simulink model "plant"  (R2024b)
settings: Solver=VariableStepAuto  StartTime=0.0  StopTime=20  RelTol=1e-3
undefined symbols (not defined in the file): Earth, init, Ts, Vehicle, WGS84
libraries: slpidlib x6, environmentLibrary x2, shared6dof x1, aerolibtransform2 x1
settings Model: Creator=Gabriel Fernandes  LastModifiedBy=Gabriel Fernandes

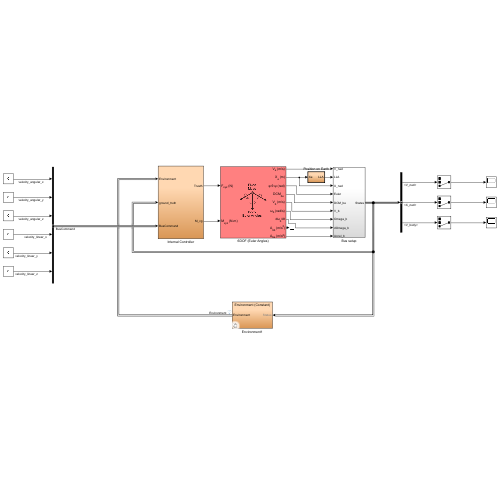
[thumbnail: Simulink's stored preview of the top-level diagram]
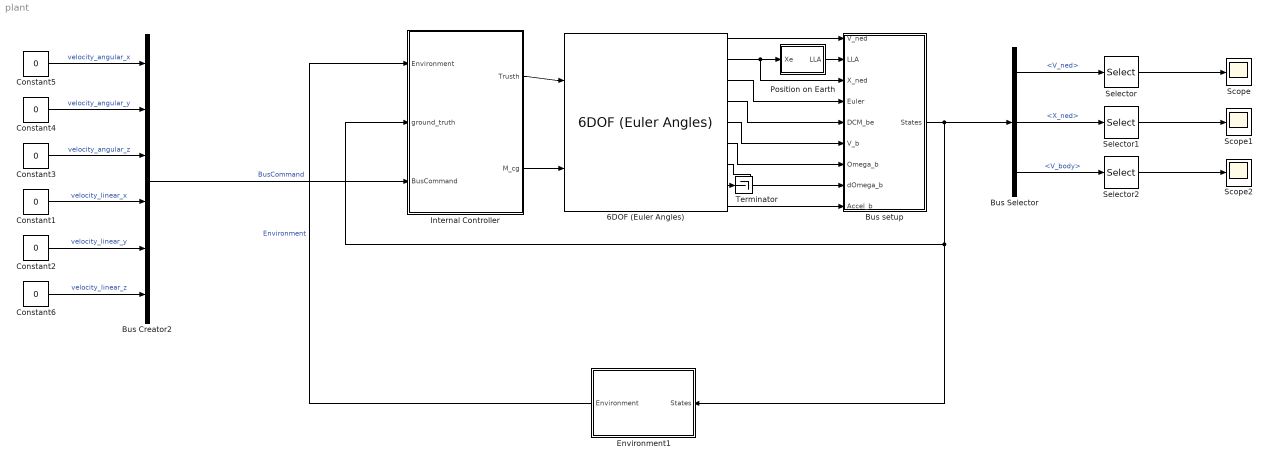
== system plant ==
  6DOF (Euler Angles) : shared6dof/6DOF (Euler Angles)  units=Metric (MKS)  mtype=Fixed  rep=Euler Angles  xme_0=init.posNED  Vm_0=init.vb  eul_0=init.euler  pm_0=init.angRates  mass_0=Vehicle.Airframe.mass  mass_e=0.5  mass_f=2.0  inertia=Vehicle.Airframe.inertia  inertia_e=eye(3)  inertia_f=2*eye(3)  k_quat=Vehicle.SixDOF.quatGain  vre_flag=on  abi_flag=on  aMode=aMode  xme_statename=''  Vm_statename=''  eul_statename=''  quat_statename=''  pm_statename=''  mass_statename=''
  Bus Creator2 : BusCreator  Inputs=6  OutDataTypeStr=Bus: BusCommand
  Bus Selector : BusSelector  OutputSignals=V_ned,X_ned,V_body
  Bus setup : Subsystem
  Constant{1..6} (6 alike) : Constant  Value=0
  Environment1 : Subsystem  Variant=on
  Internal Controller : Subsystem
  Position on Earth : Subsystem  Priority=1  TreatAsAtomicUnit=on
  Scope : Scope
  Scope1 : Scope
  Scope2 : Scope
  Selector : Selector  InputPortWidth=3  IndexOptions=Index vector (dialog)  Indices=3  OutputSizes=1
  Selector1 : Selector  InputPortWidth=3  IndexOptions=Index vector (dialog)  Indices=3  OutputSizes=1
  Selector2 : Selector  InputPortWidth=3  IndexOptions=Index vector (dialog)  Indices=3  OutputSizes=1
  Terminator : Terminator
  wires:
  6DOF (Euler Angles)/5 -> Bus setup/6(V_b)
  6DOF (Euler Angles)/2 -> Bus setup/3(X_ned), Position on Earth/1(Xe)
  6DOF (Euler Angles)/8 -> Terminator/1
  6DOF (Euler Angles)/6 -> Bus setup/7(Omega_b)
  6DOF (Euler Angles)/3 -> Bus setup/4(Euler)
  Position on Earth/1(LLA) -> Bus setup/2(LLA)
  6DOF (Euler Angles)/1 -> Bus setup/1(V_ned)
  6DOF (Euler Angles)/7 -> Bus setup/8(dOmega_b)
  6DOF (Euler Angles)/9 -> Bus setup/9(Accel_b)
  6DOF (Euler Angles)/4 -> Bus setup/5(DCM_be)
  Internal Controller/1(Trusth) -> 6DOF (Euler Angles)/1
  Internal Controller/2(M_cg) -> 6DOF (Euler Angles)/2
  Bus setup/1(States) -> Environment1/1(States), Internal Controller/2(ground_truth), Bus Selector/1
  Environment1/1(Environment) -> Internal Controller/1(Environment)  "Environment"
  Constant3/1 -> Bus Creator2/3  "velocity_angular_z"
  Constant5/1 -> Bus Creator2/1  "velocity_angular_x"
  Constant4/1 -> Bus Creator2/2  "velocity_angular_y"
  Constant1/1 -> Bus Creator2/4  "velocity_linear_x"
  Constant2/1 -> Bus Creator2/5  "velocity_linear_y"
  Constant6/1 -> Bus Creator2/6  "velocity_linear_z"
  Bus Creator2/1 -> Internal Controller/3(BusCommand)  "BusCommand"
  Bus Selector/1 -> Selector/1  "<V_ned>"
  Bus Selector/2 -> Selector1/1  "<X_ned>"
  Bus Selector/3 -> Selector2/1  "<V_body>"
  Selector/1 -> Scope/1
  Selector1/1 -> Scope1/1
  Selector2/1 -> Scope2/1

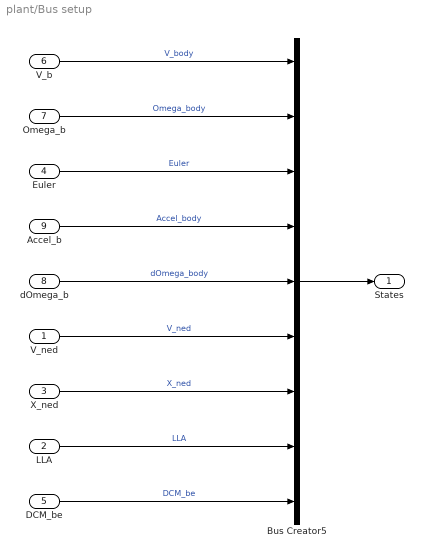
== system plant/Bus setup ==
  V_ned : Inport  Unit=m/second  PortDimensions=3
  LLA : Inport  Port=2  PortDimensions=3
  X_ned : Inport  Port=3  Unit=m  PortDimensions=3
  Euler : Inport  Port=4  Unit=rad  PortDimensions=3
  DCM_be : Inport  Port=5  PortDimensions=[3 3]
  V_b : Inport  Port=6  Unit=m/s  PortDimensions=3
  Omega_b : Inport  Port=7  Unit=rad/s  PortDimensions=3
  dOmega_b : Inport  Port=8  Unit=rad/s^2  PortDimensions=3
  Accel_b : Inport  Port=9  Unit=m/s^2  PortDimensions=3
  Bus Creator5 : BusCreator  Inputs=9  OutDataTypeStr=Bus: StatesBus  NonVirtualBus=on
  States : Outport  VectorParamsAs1DForOutWhenUnconnected=off
  wires:
  Bus Creator5/1 -> States/1
  V_b/1 -> Bus Creator5/1  "V_body"
  Omega_b/1 -> Bus Creator5/2  "Omega_body"
  Euler/1 -> Bus Creator5/3  "Euler"
  X_ned/1 -> Bus Creator5/7  "X_ned"
  Accel_b/1 -> Bus Creator5/4  "Accel_body"
  LLA/1 -> Bus Creator5/8  "LLA"
  dOmega_b/1 -> Bus Creator5/5  "dOmega_body"
  DCM_be/1 -> Bus Creator5/9  "DCM_be"
  V_ned/1 -> Bus Creator5/6  "V_ned"

== system plant/Environment1 ==
  note: VSS_ENVIRONMENT = 0 will select constant environment variables
      | VSS_ENVIRONMENT = 1 will select environment variables depending on position
  States : Inport  OutDataTypeStr=Bus: StatesBus
  Environment (Constant) : environmentLibrary/Environment (Constant)  SystemSampleTime=-1  VariantControl=VSS_ENVIRONMENT==EnvironmentMode.Constant  VariantActivationTime=update diagram  AllowFlexibleInterface=on  Latency=0  AutoFrameSizeCalculation=off
  Environment (Variable) : environmentLibrary/Environment (Variable)  SystemSampleTime=-1  VariantControl=VSS_ENVIRONMENT==EnvironmentMode.Variable  VariantActivationTime=update diagram  AllowFlexibleInterface=on  Latency=0  AutoFrameSizeCalculation=off
  Environment : Outport  OutDataTypeStr=Bus: EnvironmentBus  VectorParamsAs1DForOutWhenUnconnected=off

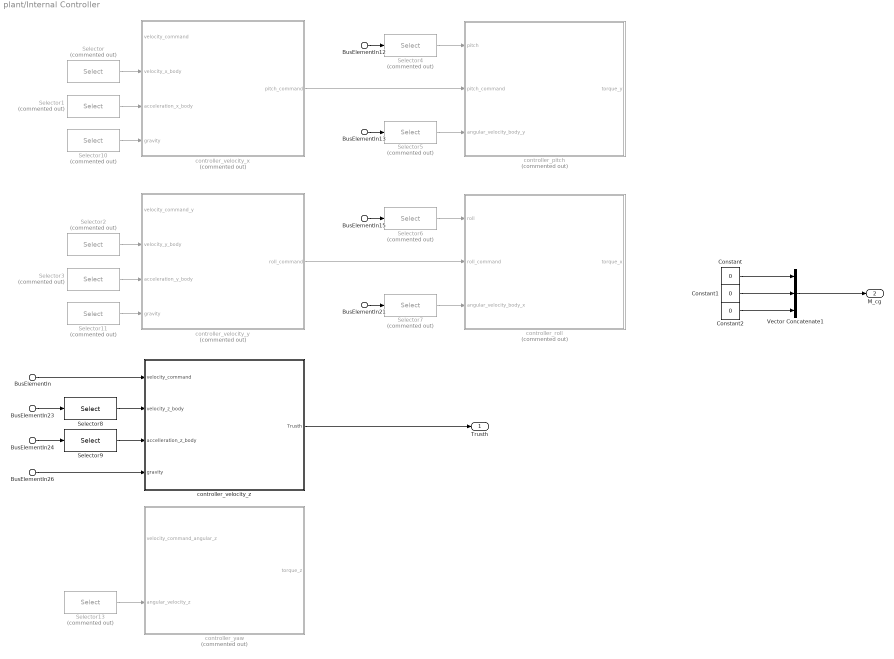
== system plant/Internal Controller ==
  BusElementIn26 : Inport  PortName=Environment  Element=Gravity_ned
  BusElementIn23 : Inport  Port=2  PortName=ground_truth  Element=V_body
  BusElementIn13 : Inport  Port=2  PortName=ground_truth  Element=Omega_body
  BusElementIn12 : Inport  Port=2  PortName=ground_truth  Element=Euler
  BusElementIn15 : Inport  Port=2  PortName=ground_truth  Element=Euler
  BusElementIn21 : Inport  Port=2  PortName=ground_truth  Element=Accel_body
  BusElementIn24 : Inport  Port=2  PortName=ground_truth  Element=Accel_body
  BusElementIn : Inport  Port=3  PortName=BusCommand  Element=velocity_linear_z
  Constant : Constant  Value=0
  Constant1 : Constant  Value=0
  Constant2 : Constant  Value=0
  Selector{,1,6..7} (4 alike) : Selector  Commented=on  InputPortWidth=3  IndexOptions=Index vector (dialog)  Indices=1  OutputSizes=1
  Selector10 : Selector  Commented=on  InputPortWidth=3  IndexOptions=Index vector (dialog)  Indices=3  OutputSizes=1
  Selector11 : Selector  Commented=on  InputPortWidth=3  IndexOptions=Index vector (dialog)  Indices=3  OutputSizes=1
  Selector13 : Selector  Commented=on  InputPortWidth=3  IndexOptions=Index vector (dialog)  Indices=3  OutputSizes=1
  Selector{2..5} (4 alike) : Selector  Commented=on  InputPortWidth=3  IndexOptions=Index vector (dialog)  Indices=2  OutputSizes=1
  Selector8 : Selector  InputPortWidth=3  IndexOptions=Index vector (dialog)  Indices=3  OutputSizes=1
  Selector9 : Selector  InputPortWidth=3  IndexOptions=Index vector (dialog)  Indices=3  OutputSizes=1
  Vector Concatenate1 : Concatenate  NumInputs=3
  controller_pitch : Subsystem  Commented=on
  controller_roll : Subsystem  Commented=on
  controller_velocity_x : Subsystem  Commented=on
  controller_velocity_y : Subsystem  Commented=on
  controller_velocity_z : Subsystem
  controller_yaw : Subsystem  Commented=on
  Trusth : Outport  Unit=N  VectorParamsAs1DForOutWhenUnconnected=off
  M_cg : Outport  Port=2  Unit=N*m  VectorParamsAs1DForOutWhenUnconnected=off
  wires:
  Vector Concatenate1/1 -> M_cg/1
  ? -> Selector/1
  Selector/1 -> controller_velocity_x/2(velocity_x_body)
  ? -> Selector1/1
  Selector1/1 -> controller_velocity_x/3(acceleration_x_body)
  ? -> Selector10/1
  ? -> Selector3/1
  ? -> Selector2/1
  Selector2/1 -> controller_velocity_y/2(velocity_y_body)
  Selector3/1 -> controller_velocity_y/3(acceleration_y_body)
  ? -> Selector11/1
  controller_velocity_x/1(pitch_command) -> controller_pitch/2(pitch_command)
  BusElementIn12/1 -> Selector4/1
  Selector4/1 -> controller_pitch/1(pitch)
  BusElementIn13/1 -> Selector5/1
  Selector5/1 -> controller_pitch/3(angular_velocity_body_y)
  Selector7/1 -> controller_roll/3(angular_velocity_body_x)
  Selector6/1 -> controller_roll/1(roll)
  controller_velocity_y/1(roll_command) -> controller_roll/2(roll_command)
  BusElementIn15/1 -> Selector6/1
  BusElementIn21/1 -> Selector7/1
  BusElementIn23/1 -> Selector8/1
  Selector8/1 -> controller_velocity_z/2(velocity_z_body)
  BusElementIn24/1 -> Selector9/1
  Selector9/1 -> controller_velocity_z/3(accelleration_z_body)
  Selector10/1 -> controller_velocity_x/4(gravity)
  Selector11/1 -> controller_velocity_y/4(gravity)
  BusElementIn26/1 -> controller_velocity_z/4(gravity)
  Selector13/1 -> controller_yaw/2(angular_velocity_z)
  controller_velocity_z/1(Trusth) -> Trusth/1
  BusElementIn/1 -> controller_velocity_z/1(velocity_command)
  Constant/1 -> Vector Concatenate1/1
  Constant1/1 -> Vector Concatenate1/2
  Constant2/1 -> Vector Concatenate1/3

== system plant/Position on Earth ==
  Xe : Inport  Unit=m
  Flat Earth to LLA : aerolibtransform2/Flat Earth to LLA  units=Metric (MKS)  ptype=Earth (WGS84)  F=1/298.257223563  R=6378137  refPosPort=off  LL0=init.posLLA(1:2)  psi=Vehicle.PositionOnEarth.FlatEarthToLLA.xAxis
  Mux : Mux  Inputs=2
  href : Constant  Value=Vehicle.PositionOnEarth.href
  LLA : Outport  VectorParamsAs1DForOutWhenUnconnected=off
  wires:
  Mux/1 -> LLA/1
  Xe/1 -> Flat Earth to LLA/1
  Flat Earth to LLA/1 -> Mux/1
  Flat Earth to LLA/2 -> Mux/2
  href/1 -> Flat Earth to LLA/2

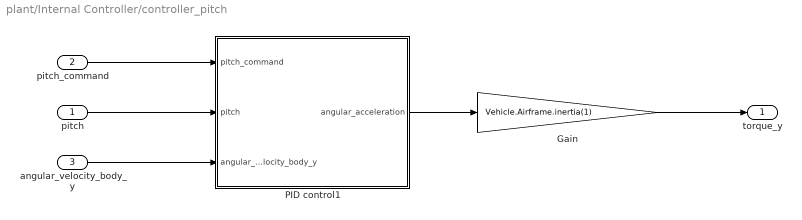
== system plant/Internal Controller/controller_pitch ==
  pitch : Inport
  pitch_command : Inport  Port=2
  angular_velocity_body_y : Inport  Port=3
  Gain : Gain  Gain=Vehicle.Airframe.inertia(1)
  PID control1 : Subsystem
  torque_y : Outport
  wires:
  pitch_command/1 -> PID control1/1(pitch_command)
  pitch/1 -> PID control1/2(pitch)
  angular_velocity_body_y/1 -> PID control1/3(angular_velocity_body_y)
  PID control1/1(angular_acceleration) -> Gain/1
  Gain/1 -> torque_y/1

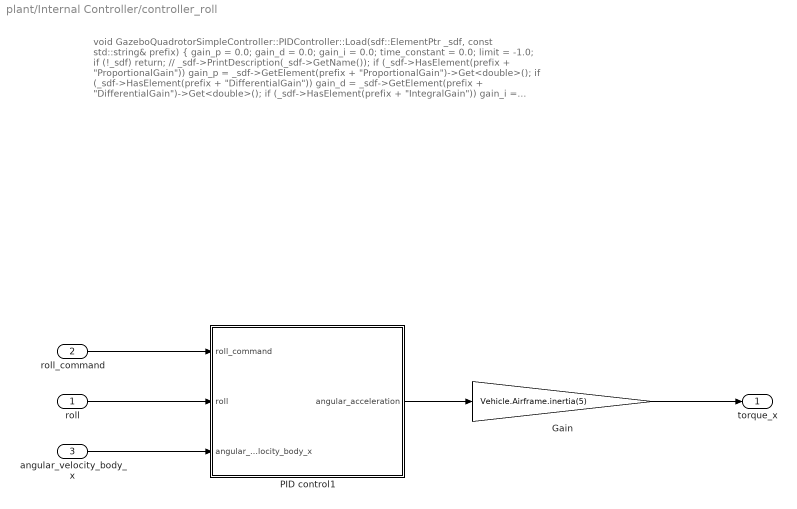
== system plant/Internal Controller/controller_roll ==
  note: void GazeboQuadrotorSimpleController::PIDController::Load(sdf::ElementPtr _sdf, const std::string& prefix)
      | {
      |   gain_p = 0.0;
      |   gain_d = 0.0;
      |   gain_i = 0.0;
      |   time_constant = 0.0;
      |   limit = -1.0;
      |
      |   if (!_sdf) return;
      |   // _sdf->PrintDescription(_sdf->GetName());
      |   if (_sdf->HasElement(prefix + "ProportionalGain")) gain_p = _sdf->GetElement(prefix + "ProportionalGain")->Get<double>();
      |   if (_sdf->HasElement(prefix + "DifferentialGain")) gain_d = _sdf->GetElement(prefix + "DifferentialGain")->Get<double>();
      |   if (_sdf->HasElement(prefix + "IntegralGain"))     gain_i = _sdf->GetElement(prefix + "IntegralGain")->Get<double>();
      |   if (_sdf->HasElement(prefix + "TimeConstant"))     time_constant = _sdf->GetElement(prefix + "TimeConstant")->Get<double>();
      |   if (_sdf->HasElement(prefix + "Limit"))            limit = _sdf->GetElement(prefix + "Limit")->Get<double>();
      | }
  roll : Inport
  roll_command : Inport  Port=2
  angular_velocity_body_x : Inport  Port=3
  Gain : Gain  Gain=Vehicle.Airframe.inertia(5)
  PID control1 : Subsystem
  torque_x : Outport
  wires:
  roll_command/1 -> PID control1/1(roll_command)
  roll/1 -> PID control1/2(roll)
  angular_velocity_body_x/1 -> PID control1/3(angular_velocity_body_x)
  PID control1/1(angular_acceleration) -> Gain/1
  Gain/1 -> torque_x/1

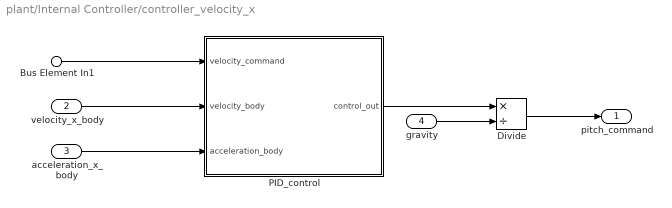
== system plant/Internal Controller/controller_velocity_x ==
  Bus Element In1 : Inport  PortName=velocity_command
  velocity_x_body : Inport  Port=2
  acceleration_x_body : Inport  Port=3
  gravity : Inport  Port=4
  Divide : Product  Inputs=*/
  PID_control : Subsystem
  pitch_command : Outport
  wires:
  velocity_x_body/1 -> PID_control/2(velocity_body)
  acceleration_x_body/1 -> PID_control/3(acceleration_body)
  PID_control/1(control_out) -> Divide/1
  Divide/1 -> pitch_command/1
  gravity/1 -> Divide/2
  Bus Element In1/1 -> PID_control/1(velocity_command)

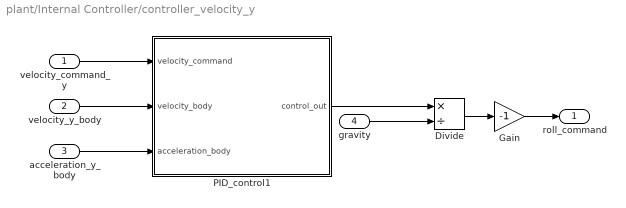
== system plant/Internal Controller/controller_velocity_y ==
  velocity_command_y : Inport
  velocity_y_body : Inport  Port=2
  acceleration_y_body : Inport  Port=3
  gravity : Inport  Port=4
  Divide : Product  Inputs=*/
  Gain : Gain  Gain=-1
  PID_control1 : Subsystem
  roll_command : Outport
  wires:
  PID_control1/1(control_out) -> Divide/1
  gravity/1 -> Divide/2
  velocity_command_y/1 -> PID_control1/1(velocity_command)
  velocity_y_body/1 -> PID_control1/2(velocity_body)
  acceleration_y_body/1 -> PID_control1/3(acceleration_body)
  Divide/1 -> Gain/1
  Gain/1 -> roll_command/1

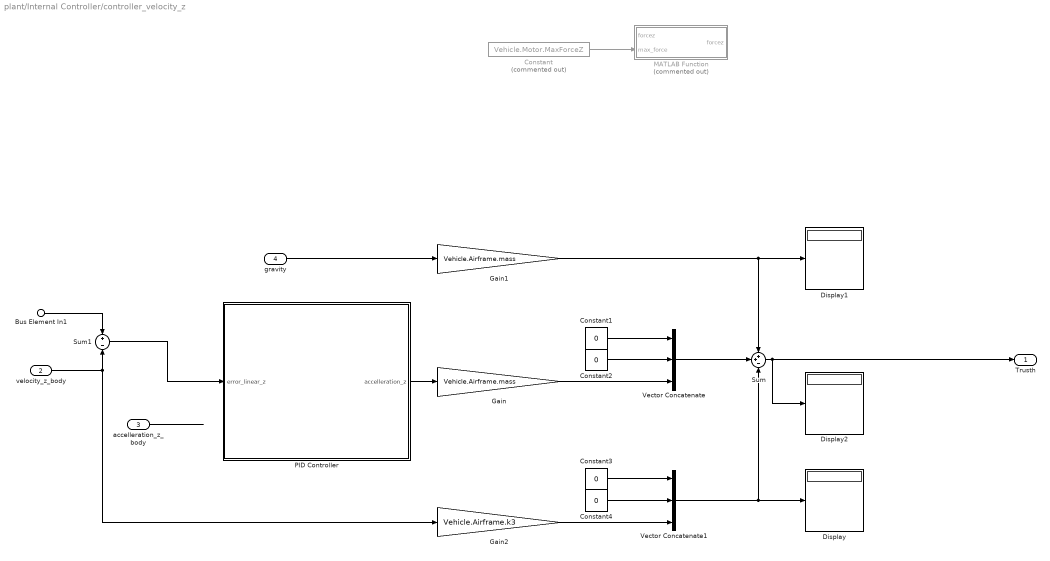
== system plant/Internal Controller/controller_velocity_z ==
  Bus Element In1 : Inport  PortName=velocity_command
  velocity_z_body : Inport  Port=2
  accelleration_z_body : Inport  Port=3
  gravity : Inport  Port=4
  Constant : Constant  Commented=on  Value=Vehicle.Motor.MaxForceZ
  Constant{1..4} (4 alike) : Constant  Value=0
  Display : Display
  Display1 : Display
  Display2 : Display
  Gain : Gain  Gain=Vehicle.Airframe.mass
  Gain1 : Gain  Gain=Vehicle.Airframe.mass
  Gain2 : Gain  Gain=Vehicle.Airframe.k3
  MATLAB Function : MATLAB Function  Commented=on  TreatAsAtomicUnit=on
  PID Controller : Subsystem
  Sum : Sum  Inputs=++-
  Sum1 : Sum  Inputs=+-
  Vector Concatenate : Concatenate  NumInputs=3
  Vector Concatenate1 : Concatenate  NumInputs=3
  Trusth : Outport
  wires:
  Sum/1 -> Display2/1, Trusth/1
  gravity/1 -> Gain1/1
  Bus Element In1/1 -> Sum1/1
  velocity_z_body/1 -> Gain2/1, Sum1/2
  accelleration_z_body/1 -> ?
  PID Controller/1(accelleration_z) -> Gain/1
  Gain1/1 -> Sum/1, Display1/1
  Gain/1 -> Vector Concatenate/3
  Vector Concatenate/1 -> Sum/2
  Constant1/1 -> Vector Concatenate/1
  Constant2/1 -> Vector Concatenate/2
  ? -> MATLAB Function/1("forcez ")
  Constant/1 -> MATLAB Function/2(max_force)
  Gain2/1 -> Vector Concatenate1/3
  Sum1/1 -> PID Controller/1(error_linear_z)
  Constant3/1 -> Vector Concatenate1/1
  Constant4/1 -> Vector Concatenate1/2
  Vector Concatenate1/1 -> Display/1, Sum/3

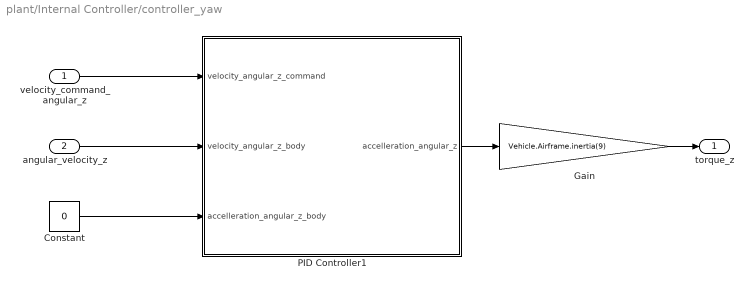
== system plant/Internal Controller/controller_yaw ==
  velocity_command_angular_z : Inport
  angular_velocity_z : Inport  Port=2
  Constant : Constant  Value=0
  Gain : Gain  Gain=Vehicle.Airframe.inertia(9)
  PID Controller1 : Subsystem
  torque_z : Outport
  wires:
  velocity_command_angular_z/1 -> PID Controller1/1(velocity_angular_z_command)
  angular_velocity_z/1 -> PID Controller1/2(velocity_angular_z_body)
  Constant/1 -> PID Controller1/3(accelleration_angular_z_body)
  PID Controller1/1(accelleration_angular_z) -> Gain/1
  Gain/1 -> torque_z/1

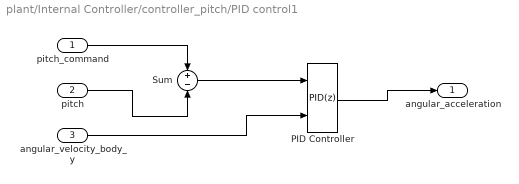
== system plant/Internal Controller/controller_pitch/PID control1 ==
  pitch_command : Inport
  pitch : Inport  Port=2
  angular_velocity_body_y : Inport  Port=3
  PID Controller : slpidlib/PID Controller  Controller=PID  Form=Parallel  TimeDomain=Discrete-time  UseExternalTs=off  SampleTime=Ts  IntegratorMethod=Forward Euler  FilterMethod=Forward Euler  ControllerParametersSource=internal  P=1  I=1  UseKiTs=off  D=0  UseExternalDerivativeSource=on  N=100  UseFilter=on  TunerSelectOption=Transfer Function Based (PID Tuner App)  InitialConditionSource=internal  InitialConditionForIntegrator=0  InitialConditionForFilter=0  DifferentiatorICPrevScaledInput=0  ExternalReset=none  TrackingMode=off  Kt=1  LimitOutput=off  SatLimitsSource=internal  UpperSaturationLimit=inf  LowerSaturationLimit=-inf  LinearizeAsGain=on  AntiWindupMode=none  Kb=1  LimitIntegrator=off  UpperIntegratorSaturationLimit=inf  LowerIntegratorSaturationLimit=-inf  POutMin=[]  POutMax=[]  IOutMin=[]  IOutMax=[]  DOutMin=[]  DOutMax=[]  NOutMin=[]  NOutMax=[]  SumOutMin=[]  SumOutMax=[]  SaturationOutMin=[]  SaturationOutMax=[]  PParamMin=[]  PParamMax=[]  IParamMin=[]  IParamMax=[]  DParamMin=[]  DParamMax=[]  NParamMin=[]  NParamMax=[]  KbParamMin=[]  KbParamMax=[]  KtParamMin=[]  KtParamMax=[]  KbOutMin=[]  KbOutMax=[]  KtOutMin=[]  KtOutMax=[]  IntegratorOutMin=[]  IntegratorOutMax=[]  FilterOutMin=[]  FilterOutMax=[]  SumI1OutMin=[]  SumI1OutMax=[]  SumI2OutMin=[]  SumI2OutMax=[]  SumI3OutMin=[]  SumI3OutMax=[]  SumI4OutMin=[]  SumI4OutMax=[]  SumDOutMin=[]  SumDOutMax=[]  DifferentiatorOutMin=[]  DifferentiatorOutMax=[]  FilterDiffOutCoefMin=[]  FilterDiffOutCoefMax=[]  ReciprocalOutMin=[]  ReciprocalOutMax=[]  SumDenOutMin=[]  SumDenOutMax=[]  SumNumOutMin=[]  SumNumOutMax=[]  DivideOutMin=[]  DivideOutMax=[]  UdiffTsProdOutMin=[]  UdiffTsProdOutMax=[]  NTsProdOutMin=[]  NTsProdOutMax=[]  UintegralTsProdOutMin=[]  UintegralTsProdOutMax=[]  UngainTsProdOutMin=[]  UngainTsProdOutMax=[]  ClampingZeroOutDataTypeStr=Inherit: Inherit via back propagation  ClampingZeroOutMin=[]  ClampingZeroOutMax=[]  FilterDenConstantOutDataTypeStr=Inherit: Inherit via back propagation  FilterDenConstantOutMin=[]  FilterDenConstantOutMax=[]  PCopyOutDataTypeStr=Inherit: Inherit via back propagation  PCopyOutMin=[]  PCopyOutMax=[]  NCopyOutDataTypeStr=Inherit: Inherit via back propagation  NCopyOutMin=[]  NCopyOutMax=[]  IntegratorContinuousStateAttributes=''  IntegratorStateMustResolveToSignalObject=off  IntegratorRTWStateStorageClass=Auto  FilterContinuousStateAttributes=''  FilterStateMustResolveToSignalObject=off  FilterRTWStateStorageClass=Auto  ParallelPVariant=InternalParameters  IdealPVariant=Disabled  IVariant=InternalParameters  DVariant=InternalParameters  IntegratorVariant=Discrete  SatVariant=Disabled  AWVariant=Passthrough  PCopyVariant=Disabled  TRVariant=Disabled  FdbkBlocksVariant=Forward  IdealPFdbkVariant=Disabled  SatFdbkVariant=Disabled  DerivativeFilterVariant=ForwardEulerFilterOnly  NVariant=InternalParameters  NCopyVariant=Disabled  FilterICVariant=InternalICsFilter  IntegratorICVariant=InternalICs  ExternalResetVariant=Disabled  TRSumVariant=Passthrough  SumFdbkVariant=Disabled  SumVariant=Sum_PID  TsampFilterVariant=InternalTs  TsampNgainVariant=Passthrough  TsampIntegralVariant=Disabled_SignalSpec  ExternalSaturationOutDataTypeStr=Inherit: Same as second input  DerivativeSourceVariant=ExternalYdot  PreIntVariant=InternalPreInt
  Sum : Sum  Inputs=+-
  angular_acceleration : Outport
  wires:
  pitch/1 -> Sum/2
  pitch_command/1 -> Sum/1
  PID Controller/1 -> angular_acceleration/1
  Sum/1 -> PID Controller/1
  angular_velocity_body_y/1 -> PID Controller/2

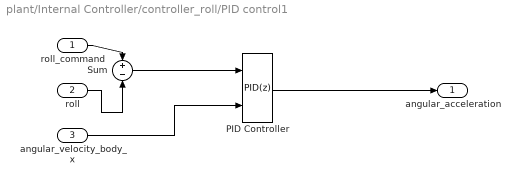
== system plant/Internal Controller/controller_roll/PID control1 ==
  roll_command : Inport
  roll : Inport  Port=2
  angular_velocity_body_x : Inport  Port=3
  PID Controller : slpidlib/PID Controller  Controller=PID  Form=Parallel  TimeDomain=Discrete-time  UseExternalTs=off  SampleTime=Ts  IntegratorMethod=Forward Euler  FilterMethod=Forward Euler  ControllerParametersSource=internal  P=1  I=1  UseKiTs=off  D=0  UseExternalDerivativeSource=on  N=100  UseFilter=on  TunerSelectOption=Transfer Function Based (PID Tuner App)  InitialConditionSource=internal  InitialConditionForIntegrator=0  InitialConditionForFilter=0  DifferentiatorICPrevScaledInput=0  ExternalReset=none  TrackingMode=off  Kt=1  LimitOutput=off  SatLimitsSource=internal  UpperSaturationLimit=inf  LowerSaturationLimit=-inf  LinearizeAsGain=on  AntiWindupMode=none  Kb=1  LimitIntegrator=off  UpperIntegratorSaturationLimit=inf  LowerIntegratorSaturationLimit=-inf  POutMin=[]  POutMax=[]  IOutMin=[]  IOutMax=[]  DOutMin=[]  DOutMax=[]  NOutMin=[]  NOutMax=[]  SumOutMin=[]  SumOutMax=[]  SaturationOutMin=[]  SaturationOutMax=[]  PParamMin=[]  PParamMax=[]  IParamMin=[]  IParamMax=[]  DParamMin=[]  DParamMax=[]  NParamMin=[]  NParamMax=[]  KbParamMin=[]  KbParamMax=[]  KtParamMin=[]  KtParamMax=[]  KbOutMin=[]  KbOutMax=[]  KtOutMin=[]  KtOutMax=[]  IntegratorOutMin=[]  IntegratorOutMax=[]  FilterOutMin=[]  FilterOutMax=[]  SumI1OutMin=[]  SumI1OutMax=[]  SumI2OutMin=[]  SumI2OutMax=[]  SumI3OutMin=[]  SumI3OutMax=[]  SumI4OutMin=[]  SumI4OutMax=[]  SumDOutMin=[]  SumDOutMax=[]  DifferentiatorOutMin=[]  DifferentiatorOutMax=[]  FilterDiffOutCoefMin=[]  FilterDiffOutCoefMax=[]  ReciprocalOutMin=[]  ReciprocalOutMax=[]  SumDenOutMin=[]  SumDenOutMax=[]  SumNumOutMin=[]  SumNumOutMax=[]  DivideOutMin=[]  DivideOutMax=[]  UdiffTsProdOutMin=[]  UdiffTsProdOutMax=[]  NTsProdOutMin=[]  NTsProdOutMax=[]  UintegralTsProdOutMin=[]  UintegralTsProdOutMax=[]  UngainTsProdOutMin=[]  UngainTsProdOutMax=[]  ClampingZeroOutDataTypeStr=Inherit: Inherit via back propagation  ClampingZeroOutMin=[]  ClampingZeroOutMax=[]  FilterDenConstantOutDataTypeStr=Inherit: Inherit via back propagation  FilterDenConstantOutMin=[]  FilterDenConstantOutMax=[]  PCopyOutDataTypeStr=Inherit: Inherit via back propagation  PCopyOutMin=[]  PCopyOutMax=[]  NCopyOutDataTypeStr=Inherit: Inherit via back propagation  NCopyOutMin=[]  NCopyOutMax=[]  IntegratorContinuousStateAttributes=''  IntegratorStateMustResolveToSignalObject=off  IntegratorRTWStateStorageClass=Auto  FilterContinuousStateAttributes=''  FilterStateMustResolveToSignalObject=off  FilterRTWStateStorageClass=Auto  ParallelPVariant=InternalParameters  IdealPVariant=Disabled  IVariant=InternalParameters  DVariant=InternalParameters  IntegratorVariant=Discrete  SatVariant=Disabled  AWVariant=Passthrough  PCopyVariant=Disabled  TRVariant=Disabled  FdbkBlocksVariant=Forward  IdealPFdbkVariant=Disabled  SatFdbkVariant=Disabled  DerivativeFilterVariant=ForwardEulerFilterOnly  NVariant=InternalParameters  NCopyVariant=Disabled  FilterICVariant=InternalICsFilter  IntegratorICVariant=InternalICs  ExternalResetVariant=Disabled  TRSumVariant=Passthrough  SumFdbkVariant=Disabled  SumVariant=Sum_PID  TsampFilterVariant=InternalTs  TsampNgainVariant=Passthrough  TsampIntegralVariant=Disabled_SignalSpec  ExternalSaturationOutDataTypeStr=Inherit: Same as second input  DerivativeSourceVariant=ExternalYdot  PreIntVariant=InternalPreInt
  Sum : Sum  Inputs=+-
  angular_acceleration : Outport
  wires:
  roll/1 -> Sum/2
  roll_command/1 -> Sum/1
  PID Controller/1 -> angular_acceleration/1
  Sum/1 -> PID Controller/1
  angular_velocity_body_x/1 -> PID Controller/2

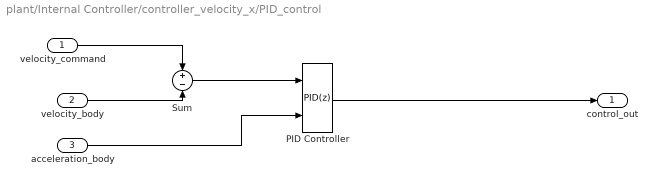
== system plant/Internal Controller/controller_velocity_x/PID_control ==
  velocity_command : Inport
  velocity_body : Inport  Port=2
  acceleration_body : Inport  Port=3
  PID Controller : slpidlib/PID Controller  Controller=PID  Form=Parallel  TimeDomain=Discrete-time  UseExternalTs=off  SampleTime=Ts  IntegratorMethod=Forward Euler  FilterMethod=Forward Euler  ControllerParametersSource=internal  P=1  I=1  UseKiTs=off  D=0  UseExternalDerivativeSource=on  N=100  UseFilter=on  TunerSelectOption=Transfer Function Based (PID Tuner App)  InitialConditionSource=internal  InitialConditionForIntegrator=0  InitialConditionForFilter=0  DifferentiatorICPrevScaledInput=0  ExternalReset=none  TrackingMode=off  Kt=1  LimitOutput=off  SatLimitsSource=internal  UpperSaturationLimit=inf  LowerSaturationLimit=-inf  LinearizeAsGain=on  AntiWindupMode=none  Kb=1  LimitIntegrator=off  UpperIntegratorSaturationLimit=inf  LowerIntegratorSaturationLimit=-inf  POutMin=[]  POutMax=[]  IOutMin=[]  IOutMax=[]  DOutMin=[]  DOutMax=[]  NOutMin=[]  NOutMax=[]  SumOutMin=[]  SumOutMax=[]  SaturationOutMin=[]  SaturationOutMax=[]  PParamMin=[]  PParamMax=[]  IParamMin=[]  IParamMax=[]  DParamMin=[]  DParamMax=[]  NParamMin=[]  NParamMax=[]  KbParamMin=[]  KbParamMax=[]  KtParamMin=[]  KtParamMax=[]  KbOutMin=[]  KbOutMax=[]  KtOutMin=[]  KtOutMax=[]  IntegratorOutMin=[]  IntegratorOutMax=[]  FilterOutMin=[]  FilterOutMax=[]  SumI1OutMin=[]  SumI1OutMax=[]  SumI2OutMin=[]  SumI2OutMax=[]  SumI3OutMin=[]  SumI3OutMax=[]  SumI4OutMin=[]  SumI4OutMax=[]  SumDOutMin=[]  SumDOutMax=[]  DifferentiatorOutMin=[]  DifferentiatorOutMax=[]  FilterDiffOutCoefMin=[]  FilterDiffOutCoefMax=[]  ReciprocalOutMin=[]  ReciprocalOutMax=[]  SumDenOutMin=[]  SumDenOutMax=[]  SumNumOutMin=[]  SumNumOutMax=[]  DivideOutMin=[]  DivideOutMax=[]  UdiffTsProdOutMin=[]  UdiffTsProdOutMax=[]  NTsProdOutMin=[]  NTsProdOutMax=[]  UintegralTsProdOutMin=[]  UintegralTsProdOutMax=[]  UngainTsProdOutMin=[]  UngainTsProdOutMax=[]  ClampingZeroOutDataTypeStr=Inherit: Inherit via back propagation  ClampingZeroOutMin=[]  ClampingZeroOutMax=[]  FilterDenConstantOutDataTypeStr=Inherit: Inherit via back propagation  FilterDenConstantOutMin=[]  FilterDenConstantOutMax=[]  PCopyOutDataTypeStr=Inherit: Inherit via back propagation  PCopyOutMin=[]  PCopyOutMax=[]  NCopyOutDataTypeStr=Inherit: Inherit via back propagation  NCopyOutMin=[]  NCopyOutMax=[]  IntegratorContinuousStateAttributes=''  IntegratorStateMustResolveToSignalObject=off  IntegratorRTWStateStorageClass=Auto  FilterContinuousStateAttributes=''  FilterStateMustResolveToSignalObject=off  FilterRTWStateStorageClass=Auto  ParallelPVariant=InternalParameters  IdealPVariant=Disabled  IVariant=InternalParameters  DVariant=InternalParameters  IntegratorVariant=Discrete  SatVariant=Disabled  AWVariant=Passthrough  PCopyVariant=Disabled  TRVariant=Disabled  FdbkBlocksVariant=Forward  IdealPFdbkVariant=Disabled  SatFdbkVariant=Disabled  DerivativeFilterVariant=ForwardEulerFilterOnly  NVariant=InternalParameters  NCopyVariant=Disabled  FilterICVariant=InternalICsFilter  IntegratorICVariant=InternalICs  ExternalResetVariant=Disabled  TRSumVariant=Passthrough  SumFdbkVariant=Disabled  SumVariant=Sum_PID  TsampFilterVariant=InternalTs  TsampNgainVariant=Passthrough  TsampIntegralVariant=Disabled_SignalSpec  ExternalSaturationOutDataTypeStr=Inherit: Same as second input  DerivativeSourceVariant=ExternalYdot  PreIntVariant=InternalPreInt
  Sum : Sum  Inputs=+-
  control_out : Outport
  wires:
  velocity_body/1 -> Sum/2
  velocity_command/1 -> Sum/1
  PID Controller/1 -> control_out/1
  Sum/1 -> PID Controller/1
  acceleration_body/1 -> PID Controller/2

== system plant/Internal Controller/controller_velocity_y/PID_control1 ==
  velocity_command : Inport
  velocity_body : Inport  Port=2
  acceleration_body : Inport  Port=3
  PID Controller : slpidlib/PID Controller  Controller=PID  Form=Parallel  TimeDomain=Discrete-time  UseExternalTs=off  SampleTime=Ts  IntegratorMethod=Forward Euler  FilterMethod=Forward Euler  ControllerParametersSource=internal  P=1  I=1  UseKiTs=off  D=0  UseExternalDerivativeSource=on  N=100  UseFilter=on  TunerSelectOption=Transfer Function Based (PID Tuner App)  InitialConditionSource=internal  InitialConditionForIntegrator=0  InitialConditionForFilter=0  DifferentiatorICPrevScaledInput=0  ExternalReset=none  TrackingMode=off  Kt=1  LimitOutput=off  SatLimitsSource=internal  UpperSaturationLimit=inf  LowerSaturationLimit=-inf  LinearizeAsGain=on  AntiWindupMode=none  Kb=1  LimitIntegrator=off  UpperIntegratorSaturationLimit=inf  LowerIntegratorSaturationLimit=-inf  POutMin=[]  POutMax=[]  IOutMin=[]  IOutMax=[]  DOutMin=[]  DOutMax=[]  NOutMin=[]  NOutMax=[]  SumOutMin=[]  SumOutMax=[]  SaturationOutMin=[]  SaturationOutMax=[]  PParamMin=[]  PParamMax=[]  IParamMin=[]  IParamMax=[]  DParamMin=[]  DParamMax=[]  NParamMin=[]  NParamMax=[]  KbParamMin=[]  KbParamMax=[]  KtParamMin=[]  KtParamMax=[]  KbOutMin=[]  KbOutMax=[]  KtOutMin=[]  KtOutMax=[]  IntegratorOutMin=[]  IntegratorOutMax=[]  FilterOutMin=[]  FilterOutMax=[]  SumI1OutMin=[]  SumI1OutMax=[]  SumI2OutMin=[]  SumI2OutMax=[]  SumI3OutMin=[]  SumI3OutMax=[]  SumI4OutMin=[]  SumI4OutMax=[]  SumDOutMin=[]  SumDOutMax=[]  DifferentiatorOutMin=[]  DifferentiatorOutMax=[]  FilterDiffOutCoefMin=[]  FilterDiffOutCoefMax=[]  ReciprocalOutMin=[]  ReciprocalOutMax=[]  SumDenOutMin=[]  SumDenOutMax=[]  SumNumOutMin=[]  SumNumOutMax=[]  DivideOutMin=[]  DivideOutMax=[]  UdiffTsProdOutMin=[]  UdiffTsProdOutMax=[]  NTsProdOutMin=[]  NTsProdOutMax=[]  UintegralTsProdOutMin=[]  UintegralTsProdOutMax=[]  UngainTsProdOutMin=[]  UngainTsProdOutMax=[]  ClampingZeroOutDataTypeStr=Inherit: Inherit via back propagation  ClampingZeroOutMin=[]  ClampingZeroOutMax=[]  FilterDenConstantOutDataTypeStr=Inherit: Inherit via back propagation  FilterDenConstantOutMin=[]  FilterDenConstantOutMax=[]  PCopyOutDataTypeStr=Inherit: Inherit via back propagation  PCopyOutMin=[]  PCopyOutMax=[]  NCopyOutDataTypeStr=Inherit: Inherit via back propagation  NCopyOutMin=[]  NCopyOutMax=[]  IntegratorContinuousStateAttributes=''  IntegratorStateMustResolveToSignalObject=off  IntegratorRTWStateStorageClass=Auto  FilterContinuousStateAttributes=''  FilterStateMustResolveToSignalObject=off  FilterRTWStateStorageClass=Auto  ParallelPVariant=InternalParameters  IdealPVariant=Disabled  IVariant=InternalParameters  DVariant=InternalParameters  IntegratorVariant=Discrete  SatVariant=Disabled  AWVariant=Passthrough  PCopyVariant=Disabled  TRVariant=Disabled  FdbkBlocksVariant=Forward  IdealPFdbkVariant=Disabled  SatFdbkVariant=Disabled  DerivativeFilterVariant=ForwardEulerFilterOnly  NVariant=InternalParameters  NCopyVariant=Disabled  FilterICVariant=InternalICsFilter  IntegratorICVariant=InternalICs  ExternalResetVariant=Disabled  TRSumVariant=Passthrough  SumFdbkVariant=Disabled  SumVariant=Sum_PID  TsampFilterVariant=InternalTs  TsampNgainVariant=Passthrough  TsampIntegralVariant=Disabled_SignalSpec  ExternalSaturationOutDataTypeStr=Inherit: Same as second input  DerivativeSourceVariant=ExternalYdot  PreIntVariant=InternalPreInt
  Sum : Sum  Inputs=+-
  control_out : Outport
  wires:
  velocity_body/1 -> Sum/2
  velocity_command/1 -> Sum/1
  PID Controller/1 -> control_out/1
  Sum/1 -> PID Controller/1
  acceleration_body/1 -> PID Controller/2

== system plant/Internal Controller/controller_velocity_z/PID Controller ==
  error_linear_z : Inport
  PID Controller1 : slpidlib/PID Controller  Controller=PID  Form=Parallel  TimeDomain=Discrete-time  UseExternalTs=off  SampleTime=Ts  IntegratorMethod=Forward Euler  FilterMethod=Forward Euler  ControllerParametersSource=internal  P=5.19512309350094  I=9.18093929355307  UseKiTs=off  D=0.0129304268631676  UseExternalDerivativeSource=off  N=1.71307818629578  UseFilter=off  TunerSelectOption=Transfer Function Based (PID Tuner App)  InitialConditionSource=internal  InitialConditionForIntegrator=0  InitialConditionForFilter=0  DifferentiatorICPrevScaledInput=0  ExternalReset=none  TrackingMode=off  Kt=1  LimitOutput=off  SatLimitsSource=internal  UpperSaturationLimit=inf  LowerSaturationLimit=-inf  LinearizeAsGain=on  AntiWindupMode=none  Kb=1  LimitIntegrator=off  UpperIntegratorSaturationLimit=inf  LowerIntegratorSaturationLimit=-inf  POutMin=[]  POutMax=[]  IOutMin=[]  IOutMax=[]  DOutMin=[]  DOutMax=[]  NOutMin=[]  NOutMax=[]  SumOutMin=[]  SumOutMax=[]  SaturationOutMin=[]  SaturationOutMax=[]  PParamMin=[]  PParamMax=[]  IParamMin=[]  IParamMax=[]  DParamMin=[]  DParamMax=[]  NParamMin=[]  NParamMax=[]  KbParamMin=[]  KbParamMax=[]  KtParamMin=[]  KtParamMax=[]  KbOutMin=[]  KbOutMax=[]  KtOutMin=[]  KtOutMax=[]  IntegratorOutMin=[]  IntegratorOutMax=[]  FilterOutMin=[]  FilterOutMax=[]  SumI1OutMin=[]  SumI1OutMax=[]  SumI2OutMin=[]  SumI2OutMax=[]  SumI3OutMin=[]  SumI3OutMax=[]  SumI4OutMin=[]  SumI4OutMax=[]  SumDOutMin=[]  SumDOutMax=[]  DifferentiatorOutMin=[]  DifferentiatorOutMax=[]  FilterDiffOutCoefMin=[]  FilterDiffOutCoefMax=[]  ReciprocalOutMin=[]  ReciprocalOutMax=[]  SumDenOutMin=[]  SumDenOutMax=[]  SumNumOutMin=[]  SumNumOutMax=[]  DivideOutMin=[]  DivideOutMax=[]  UdiffTsProdOutMin=[]  UdiffTsProdOutMax=[]  NTsProdOutMin=[]  NTsProdOutMax=[]  UintegralTsProdOutMin=[]  UintegralTsProdOutMax=[]  UngainTsProdOutMin=[]  UngainTsProdOutMax=[]  ClampingZeroOutDataTypeStr=Inherit: Inherit via back propagation  ClampingZeroOutMin=[]  ClampingZeroOutMax=[]  FilterDenConstantOutDataTypeStr=Inherit: Inherit via back propagation  FilterDenConstantOutMin=[]  FilterDenConstantOutMax=[]  PCopyOutDataTypeStr=Inherit: Inherit via back propagation  PCopyOutMin=[]  PCopyOutMax=[]  NCopyOutDataTypeStr=Inherit: Inherit via back propagation  NCopyOutMin=[]  NCopyOutMax=[]  IntegratorContinuousStateAttributes=''  IntegratorStateMustResolveToSignalObject=off  IntegratorRTWStateStorageClass=Auto  FilterContinuousStateAttributes=''  FilterStateMustResolveToSignalObject=off  FilterRTWStateStorageClass=Auto  ParallelPVariant=InternalParameters  IdealPVariant=Disabled  IVariant=InternalParameters  DVariant=InternalParameters  IntegratorVariant=Discrete  SatVariant=Disabled  AWVariant=Passthrough  PCopyVariant=Disabled  TRVariant=Disabled  FdbkBlocksVariant=Forward  IdealPFdbkVariant=Disabled  SatFdbkVariant=Disabled  DerivativeFilterVariant=Differentiator  NVariant=Passthrough  NCopyVariant=Disabled_SignalSpec  FilterICVariant=InternalICsDifferentiator  IntegratorICVariant=InternalICs  ExternalResetVariant=Disabled  TRSumVariant=Passthrough  SumFdbkVariant=Disabled  SumVariant=Sum_PID  TsampFilterVariant=InternalTs  TsampNgainVariant=Passthrough  TsampIntegralVariant=Disabled_SignalSpec  ExternalSaturationOutDataTypeStr=Inherit: Same as second input  DerivativeSourceVariant=ErrorSignal  PreIntVariant=InternalPreInt
  accelleration_z : Outport
  wires:
  PID Controller1/1 -> accelleration_z/1
  error_linear_z/1 -> PID Controller1/1

== system plant/Internal Controller/controller_yaw/PID Controller1 ==
  velocity_angular_z_command : Inport
  velocity_angular_z_body : Inport  Port=2
  accelleration_angular_z_body : Inport  Port=3
  PID Controller : slpidlib/PID Controller  Controller=PID  Form=Parallel  TimeDomain=Discrete-time  UseExternalTs=off  SampleTime=Ts  IntegratorMethod=Forward Euler  FilterMethod=Forward Euler  ControllerParametersSource=internal  P=1  I=1  UseKiTs=off  D=0  UseExternalDerivativeSource=on  N=100  UseFilter=on  TunerSelectOption=Transfer Function Based (PID Tuner App)  InitialConditionSource=internal  InitialConditionForIntegrator=0  InitialConditionForFilter=0  DifferentiatorICPrevScaledInput=0  ExternalReset=none  TrackingMode=off  Kt=1  LimitOutput=off  SatLimitsSource=internal  UpperSaturationLimit=inf  LowerSaturationLimit=-inf  LinearizeAsGain=on  AntiWindupMode=none  Kb=1  LimitIntegrator=off  UpperIntegratorSaturationLimit=inf  LowerIntegratorSaturationLimit=-inf  POutMin=[]  POutMax=[]  IOutMin=[]  IOutMax=[]  DOutMin=[]  DOutMax=[]  NOutMin=[]  NOutMax=[]  SumOutMin=[]  SumOutMax=[]  SaturationOutMin=[]  SaturationOutMax=[]  PParamMin=[]  PParamMax=[]  IParamMin=[]  IParamMax=[]  DParamMin=[]  DParamMax=[]  NParamMin=[]  NParamMax=[]  KbParamMin=[]  KbParamMax=[]  KtParamMin=[]  KtParamMax=[]  KbOutMin=[]  KbOutMax=[]  KtOutMin=[]  KtOutMax=[]  IntegratorOutMin=[]  IntegratorOutMax=[]  FilterOutMin=[]  FilterOutMax=[]  SumI1OutMin=[]  SumI1OutMax=[]  SumI2OutMin=[]  SumI2OutMax=[]  SumI3OutMin=[]  SumI3OutMax=[]  SumI4OutMin=[]  SumI4OutMax=[]  SumDOutMin=[]  SumDOutMax=[]  DifferentiatorOutMin=[]  DifferentiatorOutMax=[]  FilterDiffOutCoefMin=[]  FilterDiffOutCoefMax=[]  ReciprocalOutMin=[]  ReciprocalOutMax=[]  SumDenOutMin=[]  SumDenOutMax=[]  SumNumOutMin=[]  SumNumOutMax=[]  DivideOutMin=[]  DivideOutMax=[]  UdiffTsProdOutMin=[]  UdiffTsProdOutMax=[]  NTsProdOutMin=[]  NTsProdOutMax=[]  UintegralTsProdOutMin=[]  UintegralTsProdOutMax=[]  UngainTsProdOutMin=[]  UngainTsProdOutMax=[]  ClampingZeroOutDataTypeStr=Inherit: Inherit via back propagation  ClampingZeroOutMin=[]  ClampingZeroOutMax=[]  FilterDenConstantOutDataTypeStr=Inherit: Inherit via back propagation  FilterDenConstantOutMin=[]  FilterDenConstantOutMax=[]  PCopyOutDataTypeStr=Inherit: Inherit via back propagation  PCopyOutMin=[]  PCopyOutMax=[]  NCopyOutDataTypeStr=Inherit: Inherit via back propagation  NCopyOutMin=[]  NCopyOutMax=[]  IntegratorContinuousStateAttributes=''  IntegratorStateMustResolveToSignalObject=off  IntegratorRTWStateStorageClass=Auto  FilterContinuousStateAttributes=''  FilterStateMustResolveToSignalObject=off  FilterRTWStateStorageClass=Auto  ParallelPVariant=InternalParameters  IdealPVariant=Disabled  IVariant=InternalParameters  DVariant=InternalParameters  IntegratorVariant=Discrete  SatVariant=Disabled  AWVariant=Passthrough  PCopyVariant=Disabled  TRVariant=Disabled  FdbkBlocksVariant=Forward  IdealPFdbkVariant=Disabled  SatFdbkVariant=Disabled  DerivativeFilterVariant=ForwardEulerFilterOnly  NVariant=InternalParameters  NCopyVariant=Disabled  FilterICVariant=InternalICsFilter  IntegratorICVariant=InternalICs  ExternalResetVariant=Disabled  TRSumVariant=Passthrough  SumFdbkVariant=Disabled  SumVariant=Sum_PID  TsampFilterVariant=InternalTs  TsampNgainVariant=Passthrough  TsampIntegralVariant=Disabled_SignalSpec  ExternalSaturationOutDataTypeStr=Inherit: Same as second input  DerivativeSourceVariant=ExternalYdot  PreIntVariant=InternalPreInt
  Sum : Sum  Inputs=+-
  accelleration_angular_z : Outport
  wires:
  PID Controller/1 -> accelleration_angular_z/1
  velocity_angular_z_command/1 -> Sum/1
  accelleration_angular_z_body/1 -> PID Controller/2
  velocity_angular_z_body/1 -> Sum/2
  Sum/1 -> PID Controller/1

== matlab function plant/Internal Controller/controller_velocity_z/MATLAB Function ==
  data: forcez input; forcez output; max_force input
function forcez = fcn(forcez,max_force)
      if (max_force > 0.0 && forcez(3) > max_force) 
          forcez(3) = max_force; 
      end
      if (forcez(3) < 0.0) 
          forcez(3) = 0.0;
      end
